simulink model "rtwdemo_fixptdiv"  (Simulink 7.6)
settings: Solver=FixedStepDiscrete  StartTime=0.0  StopTime=10.0  FixedStep=0.001  RelTol=1e-3  SampleTimeConstraint=STIndependent
libraries: rtwdemowidgets x1
Description:
  | Efficient Fixed-Point Operations
settings Model: Creator=The MathWorks Inc.  ExtModeAutoUpdateStatusClock=off
settings DataIOCC: SaveOutput=off  SaveTime=off
settings OptimizationCC: InlineParams=on  InlineInvariantSignals=on  PassReuseOutputArgsAs=Individual arguments  StateBitsets=on  DataBitsets=on  UseTempVars=on  ZeroExternalMemoryAtStartup=off  ZeroInternalMemoryAtStartup=off  NoFixptDivByZeroProtection=on  EfficientFloat2IntCast=on  EfficientMapNaN2IntZero=off  OptimizeModelRefInitCode=on  LifeSpan=1
settings DebuggingCC: CheckExecutionContextPreStartOutputMsg=on  CheckExecutionContextRuntimeOutputMsg=on  SolverPrmCheckMsg=none  StrictBusMsg=ErrorOnBusTreatedAsVector
settings HardwareCC: ProdIntDivRoundTo=Zero  ProdEndianess=LittleEndian  ProdHWDeviceType=Generic->32-bit Embedded Processor  TargetHWDeviceType=Generic->32-bit Embedded Processor
settings RTWCC: SystemTargetFile=ert.tlc  TemplateMakefile=ert_default_tmf  Description=RTW Embedded Coder (no auto configuration)  GenerateReport=on  RTWVerbose=off  ProcessScript=ert_make_rtw_hook  IncludeHyperlinkInReport=on  LaunchReport=on
settings CodeAppCC: ForceParamTrailComments=on  IgnoreCustomStorageClasses=off  IgnoreTestpoints=on  SimulinkDataObjDesc=on  CustomSymbolStrGlobalVar=rt$N$M  CustomSymbolStrType=$N$M  CustomSymbolStrFcn=$N$M$F  CustomSymbolStrMacro=$N$M  InsertBlockDesc=on
settings ERTTargetCC: TargetFcnLib=ansi_tfl_tmw.mat  MultiwordLength=2048  GenerateSampleERTMain=on  IncludeMdlTerminateFcn=off  SupportAbsoluteTime=off  SupportNonFinite=off  SupportComplex=off  InlinedParameterPlacement=NonHierarchical  ERTCustomFileTemplate=example_file_process.tlc  ConvertIfToSwitch=off

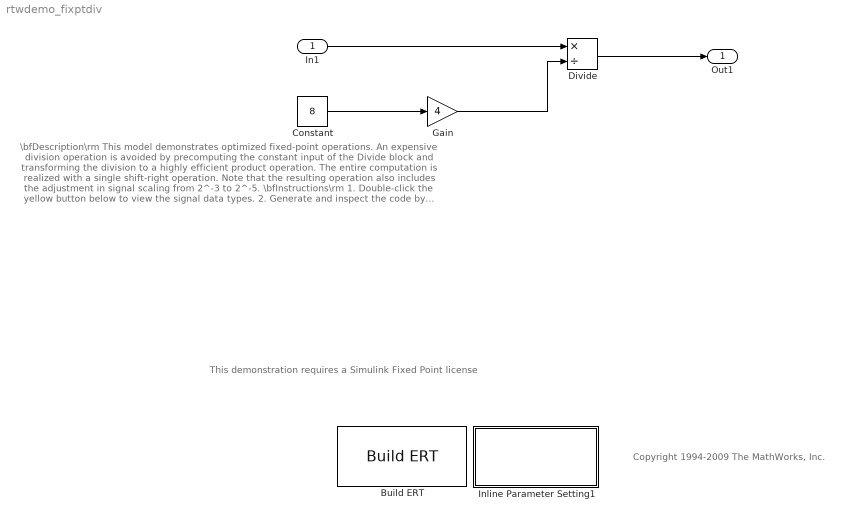
== system rtwdemo_fixptdiv ==
  note: \bfDescription\rm
      | This model demonstrates optimized fixed-point operations. An expensive division
      | operation is avoided by precomputing the constant input of the Divide block and
      | transforming the division to a highly efficient product operation. The entire
      | computation is realized with a single shift-right operation.  Note that the resulting
      | operation also includes the adjustment in signal scaling from 2^-3 to 2^-5.
      |
      | \bfInstructions\rm
      | 1. Double-click the yellow button below to view the signal data types.
      | 2. Generate and inspect the code by double-clicking the blue button below.
      |     An HTML report detailing the code is displayed automatically.
      | \bf\rm
  note: This demonstration requires a Simulink Fixed Point license
  note: Copyright 1994-2009 The MathWorks, Inc.
  In1 : Inport  OutDataTypeStr=fixdt(1,16,3)  PortDimensions=1
  Build ERT : rtwdemowidgets/Build ERT  SystemSampleTime=-1  attrib_overrides={}
  Constant : Constant  Value=8  OutDataTypeStr=Inherit: Inherit via back propagation
  Divide : Product  Inputs=*/  OutDataTypeStr=fixdt(1,16,5)
  Gain : Gain  Gain=4  OutDataTypeStr=Inherit: Inherit via back propagation
  Inline Parameter Setting1 : Subsystem
      settings: OpenFcn=m=get_param(bdroot,'name'); eval([m,'([],[],[],''compile'');']); eval([m,'([],[],[],''term'');']); clear m;
      mask Display: disp(sprintf('Display Signal\nData Types\n(double-click)'))
  Out1 : Outport
  wires:
  Divide/1 -> Out1/1
  Constant/1 -> Gain/1
  Gain/1 -> Divide/2
  In1/1 -> Divide/1

== system rtwdemo_fixptdiv/Inline Parameter Setting1 ==
